simulink library "BasicAircraftDynamicsBlock"  (R2018b)
settings: Solver=VariableStepAuto  StartTime=0.0  StopTime=10.0  RelTol=1e-3
undefined symbols (not defined in the file): ac1dyn_a_ftpss, ac1dyn_con, ac1dyn_E_ft, ac1dyn_h_ft, ac1dyn_N_ft, ac1dyn_phi_rad, ac1dyn_psi_rad, ac1dyn_theta_rad, ac1dyn_v_ftps, ac2dyn_alt0_ft, ac2dyn_lat0_rad, ac2dyn_lon0_rad, DiscIntNeverNeededParam
libraries: simulink x7
settings Model: Creator=BI28030  LastModifiedBy=BI28030

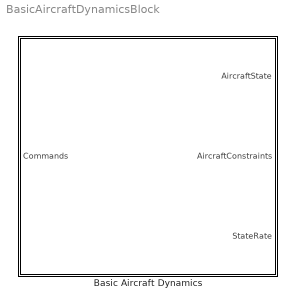
== system BasicAircraftDynamicsBlock ==
  Basic Aircraft Dynamics : Subsystem  mask(Basic Aircraft Dynamic Model){ts_dynamics=.1, v_ftps_0=ac1dyn_v_ftps, N_ft_0=ac1dyn_N_ft, E_ft_0=ac1dyn_E_ft, h_ft_0=ac1dyn_h_ft, psi_rad_0=ac1dyn_psi_rad, theta_rad_0=ac1dyn_theta_rad, phi_rad_0=ac1dyn_phi_rad, a_ftpss_0=ac1dyn_a_ftpss, v_ftps_max=ac1dyn_con.maxAirspeed_ftps, v_ftps_min=ac1dyn_con.minAirspeed_ftps, dv_ftpss_max=ac1dyn_con.maxAcceleration_ftpss, dv_ftpss_min=ac1dyn_con.minAcceleration_ftpss, dh_ftps_max=ac1dyn_con.maxVerticalRate_ftps, dh_ftps_min=ac1dyn_con.minVerticalRate_ftps, q_radps_max=ac1dyn_con.maxPitchRate_radps, phi_rad_max=ac1dyn_con.maxBankAngle_rad, dphi_radps_max=ac1dyn_con.maxRollRate_radps, r_radps_max=ac1dyn_con.maxYawRate_radps, pNUM=ac1dyn_con.dynamicsNumeratorRollRate, pDEN=ac1dyn_con.dynamicsDenominatorRollRate, hNUM=ac1dyn_con.dynamicsNumeratorVerticalRate, hDEN=ac1dyn_con.dynamicsDenominatorVerticalRate, rNUM=ac1dyn_con.dynamicsNumeratorYawRate, rDEN=ac1dyn_con.dynamicsDenominatorYawRate, lat0_rad=ac2dyn_lat0_rad, lon0_rad=ac2dyn_lon0_rad, alt_ft=ac2dyn_alt0_ft}
      mask prompts: ts_dynamics "Dynamics update parameter"; v_ftps_0 "Initial velocity (ft/s)"; N_ft_0 "Initial north position (ft)"; E_ft_0 "Initial east position (ft)"; h_ft_0 "Initial altitude (ft)"; psi_rad_0 "Initial heading (rad)"; theta_rad_0 "Initial pitch angle (rad)"; phi_rad_0 "Initial bank angle (rad)"; a_ftpss_0 "Initial acceleration (ft/s/s)"; v_ftps_max "Maximum airspeed (ft/s)"; v_ftps_min "Minimum airspeed (ft/s)"; dv_ftpss_max "Maximum acceleration (ft/s/s)"; dv_ftpss_min "Miniimum acceleration (ft/s/s)"; dh_ftps_max "Maximum vertical rate (ft/s)"; dh_ftps_min "Minimum vertical rate (ft/s)"; q_radps_max "Maximum pitch rate (rad/s)"; phi_rad_max "Maximum bank angle (rad)"; dphi_radps_max "Maximum roll rate (rad/s)"; r_radps_max "Maximum yaw rate (rad/s)"; pNUM "Roll rate discrete dynamics numerator (2x1)"; pDEN "Roll rate discrete dynamics denominator (1x1)"; hNUM "Vertical rate discrete dynamics numerator (2x1)"; hDEN "Vertical rate discrete dynamics denominator (1x1)"; rNUM "Yaw rate discrete dynamics numerator (2x1)"; rDEN "Yaw rate discrete dynamics denominator (1x1)"; lat0_rad "Latitude of ENU origin (rad)"; lon0_rad "Longitude of ENU origin (rad)"; alt_ft "Height of ENU origin (ft)"
      mask help:
      | Propagates the aircraft dynamics using 6DOF equations of motion.
      |
      | The class Simple6DOF can be used to programmatically set the parameters of Basic Aircraft Dynamics blocks.
      mask Help:
      | Propagates the aircraft dynamics using 6DOF equations of motion.
      | 
      | The class Simple6DOF can be used to programmatically set the parameters of Basic Aircraft Dynamcis blocks.
      mask DialogControl ParameterTabVar0 Prompt: Initial Conditions
      mask DialogControl ParameterTabVar01 Prompt: Constraints
      mask DialogControl ParameterTabVar012 Prompt: ENU Coordinate System

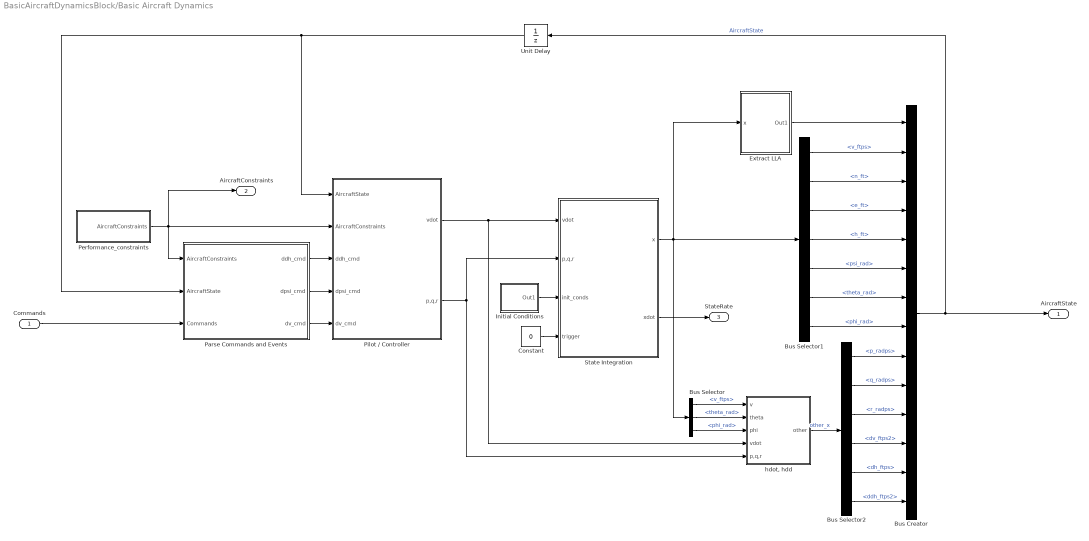
== system BasicAircraftDynamicsBlock/Basic Aircraft Dynamics ==
  Commands : Inport  OutDataTypeStr=Bus: AircraftCommands
  Bus Creator : BusCreator  Inputs=14
  Bus Selector : BusSelector  OutputSignals=v_ftps,theta_rad,phi_rad
  Bus Selector1 : BusSelector  OutputSignals=v_ftps,n_ft,e_ft,h_ft,psi_rad,theta_rad,phi_rad
  Bus Selector2 : BusSelector  OutputSignals=p_radps,q_radps,r_radps,dv_ftps2,dh_ftps,ddh_ftps2
  Constant : Constant  Value=0
  "Extract LLA " : Subsystem  mask{lat0=lat0_rad, lon0=lon0_rad, h0=alt_ft}
      mask prompts: lat0 "ENU latitude origin (rad)"; lon0 "ENU longitude origin (rad)"; h0 "ENU altitude origin (ft)"
  Initial Conditions : Subsystem
  Parse Commands and Events : Subsystem
  Performance_constraints : Subsystem
  Pilot / Controller : Subsystem
  State Integration : Subsystem
  Unit Delay : UnitDelay  SampleTime=-1
  "hdot, hdd" : Subsystem
  AircraftState : Outport  OutDataTypeStr=Bus: AircraftState
  AircraftConstraints : Outport  Port=2  OutDataTypeStr=Bus: AircraftConstraints
  StateRate : Outport  Port=3  OutDataTypeStr=Bus: AircraftStateRate
  wires:
  "Extract LLA "/1(Out1) -> Bus Creator/1
  Initial Conditions/1(Out1) -> State Integration/3(init_conds)
  Bus Selector/1 -> "hdot, hdd"/1(v)  "<v_ftps>"
  Bus Selector/2 -> "hdot, hdd"/2(theta)  "<theta_rad>"
  Bus Selector/3 -> "hdot, hdd"/3(phi)  "<phi_rad>"
  State Integration/1(x) -> Bus Selector/1, "Extract LLA "/1(x), Bus Selector1/1
  Bus Selector1/1 -> Bus Creator/2  "<v_ftps>"
  Bus Selector1/2 -> Bus Creator/3  "<n_ft>"
  Bus Selector1/3 -> Bus Creator/4  "<e_ft>"
  Bus Selector1/4 -> Bus Creator/5  "<h_ft>"
  Bus Selector1/5 -> Bus Creator/6  "<psi_rad>"
  Bus Selector1/6 -> Bus Creator/7  "<theta_rad>"
  Bus Selector1/7 -> Bus Creator/8  "<phi_rad>"
  "hdot, hdd"/1(other) -> Bus Selector2/1  "other_x"
  Bus Selector2/1 -> Bus Creator/9  "<p_radps>"
  Bus Selector2/2 -> Bus Creator/10  "<q_radps>"
  Bus Selector2/3 -> Bus Creator/11  "<r_radps>"
  Bus Selector2/4 -> Bus Creator/12  "<dv_ftps2>"
  Bus Selector2/5 -> Bus Creator/13  "<dh_ftps>"
  Bus Selector2/6 -> Bus Creator/14  "<ddh_ftps2>"
  Bus Creator/1 -> AircraftState/1, Unit Delay/1  "AircraftState"
  Constant/1 -> State Integration/4(trigger)
  Pilot / Controller/1(vdot) -> State Integration/1(vdot), "hdot, hdd"/4(vdot)
  Pilot / Controller/2(p,q,r) -> "hdot, hdd"/5(p,q,r), State Integration/2(p,q,r)
  Performance_constraints/1(AircraftConstraints) -> AircraftConstraints/1, Pilot / Controller/2(AircraftConstraints), Parse Commands and Events/1(AircraftConstraints)
  Commands/1 -> Parse Commands and Events/3(Commands)
  Parse Commands and Events/1(ddh_cmd) -> Pilot / Controller/3(ddh_cmd)
  Parse Commands and Events/2(dpsi_cmd) -> Pilot / Controller/4(dpsi_cmd)
  Parse Commands and Events/3(dv_cmd) -> Pilot / Controller/5(dv_cmd)
  Unit Delay/1 -> Pilot / Controller/1(AircraftState), Parse Commands and Events/2(AircraftState)
  State Integration/2(xdot) -> StateRate/1

== system BasicAircraftDynamicsBlock/Basic Aircraft Dynamics/Extract LLA  ==
  x : Inport
  Bus Creator1 : BusCreator  Inputs=6
  Bus Selector : BusSelector  OutputSignals=e_ft,n_ft,h_ft,v_ftps,psi_rad,theta_rad
  Constant : Constant  Value=lat0_rad
  Constant7 : Constant  Value=lon0_rad
  Constant8 : Constant  Value=alt_ft
  MATLAB Function : MATLAB Function  TreatAsAtomicUnit=on
  Out1 : Outport
  wires:
  Bus Creator1/1 -> Out1/1  "latLonAltState"
  Bus Selector/6 -> MATLAB Function/6(theta_rad)  "<theta_rad>"
  Bus Selector/5 -> MATLAB Function/5(psi_rad)  "<psi_rad>"
  Bus Selector/4 -> MATLAB Function/4(v_ftps)  "<v_ftps>"
  Bus Selector/3 -> MATLAB Function/3(u_ft)  "<h_ft>"
  Bus Selector/2 -> MATLAB Function/2(n_ft)  "<n_ft>"
  Bus Selector/1 -> MATLAB Function/1(e_ft)  "<e_ft>"
  Constant8/1 -> MATLAB Function/9(h0)
  Constant7/1 -> MATLAB Function/8(lon0)
  Constant/1 -> MATLAB Function/7(lat0)
  x/1 -> Bus Selector/1
  MATLAB Function/6(dalt_ftps) -> Bus Creator1/6  "dalt_ftps"
  MATLAB Function/5(alt_ft) -> Bus Creator1/5  "alt_ft"
  MATLAB Function/4(dlon_radps) -> Bus Creator1/4  "dlon_radps"
  MATLAB Function/3(dlat_radps) -> Bus Creator1/3  "dlat_radps"
  MATLAB Function/2(lon_rad) -> Bus Creator1/2  "lon_rad"
  MATLAB Function/1(lat_rad) -> Bus Creator1/1  "lat_rad"

== system BasicAircraftDynamicsBlock/Basic Aircraft Dynamics/Initial Conditions ==
  Bus Creator1 : BusCreator  Inputs=8
  Constant : Constant  Value=v_ftps_0
  Constant1 : Constant  Value=N_ft_0
  Constant2 : Constant  Value=E_ft_0
  Constant3 : Constant  Value=h_ft_0
  Constant4 : Constant  Value=psi_rad_0
  Constant5 : Constant  Value=theta_rad_0
  Constant6 : Constant  Value=phi_rad_0
  Constant7 : Constant  Value=a_ftpss_0
  Out1 : Outport
  wires:
  Constant1/1 -> Bus Creator1/2  "N"
  Constant2/1 -> Bus Creator1/3  "E"
  Constant3/1 -> Bus Creator1/4  "h"
  Constant4/1 -> Bus Creator1/5  "psi"
  Constant5/1 -> Bus Creator1/6  "theta"
  Constant6/1 -> Bus Creator1/7  "phi"
  Constant7/1 -> Bus Creator1/8  "a"
  Constant/1 -> Bus Creator1/1  "v"
  Bus Creator1/1 -> Out1/1

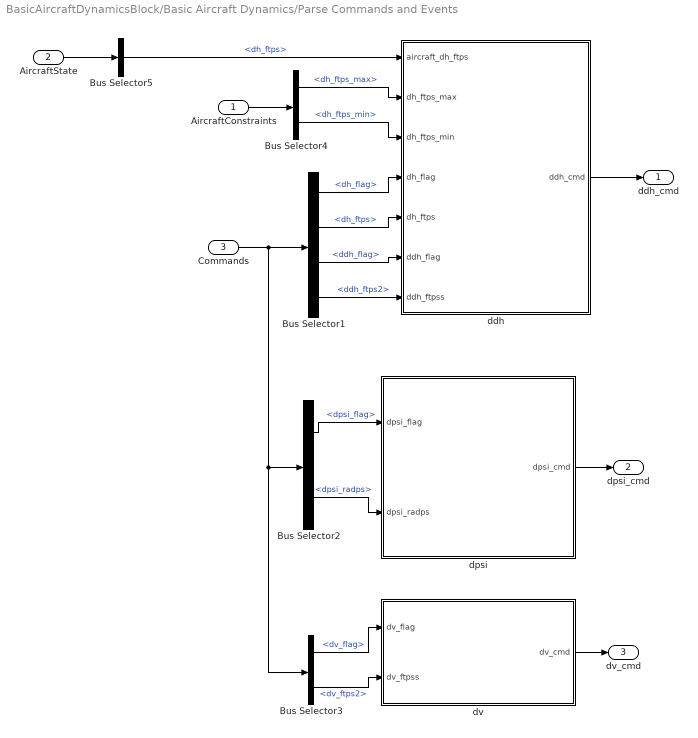
== system BasicAircraftDynamicsBlock/Basic Aircraft Dynamics/Parse Commands and Events ==
  AircraftConstraints : Inport  OutDataTypeStr=Bus: AircraftConstraints
  AircraftState : Inport  Port=2  OutDataTypeStr=Bus: AircraftState
  Commands : Inport  Port=3  OutDataTypeStr=Bus: AircraftCommands
  Bus Selector1 : BusSelector  OutputSignals=dh_flag,dh_ftps,ddh_flag,ddh_ftps2
  Bus Selector2 : BusSelector  OutputSignals=dpsi_flag,dpsi_radps
  Bus Selector3 : BusSelector  OutputSignals=dv_flag,dv_ftps2
  Bus Selector4 : BusSelector  OutputSignals=dh_ftps_max,dh_ftps_min
  Bus Selector5 : BusSelector  OutputSignals=dh_ftps
  ddh : MATLAB Function  TreatAsAtomicUnit=on
  dpsi : MATLAB Function  TreatAsAtomicUnit=on
  dv : MATLAB Function  TreatAsAtomicUnit=on
  ddh_cmd : Outport
  dpsi_cmd : Outport  Port=2
  dv_cmd : Outport  Port=3
  wires:
  dv/1(dv_cmd) -> dv_cmd/1
  dpsi/1(dpsi_cmd) -> dpsi_cmd/1
  ddh/1(ddh_cmd) -> ddh_cmd/1
  Commands/1 -> Bus Selector1/1, Bus Selector2/1, Bus Selector3/1
  Bus Selector1/1 -> ddh/4(dh_flag)  "<dh_flag>"
  Bus Selector1/2 -> ddh/5(dh_ftps)  "<dh_ftps>"
  Bus Selector1/3 -> ddh/6(ddh_flag)  "<ddh_flag>"
  Bus Selector1/4 -> ddh/7(ddh_ftpss)  "<ddh_ftps2>"
  Bus Selector2/2 -> dpsi/2(dpsi_radps)  "<dpsi_radps>"
  Bus Selector3/1 -> dv/1(dv_flag)  "<dv_flag>"
  Bus Selector3/2 -> dv/2(dv_ftpss)  "<dv_ftps2>"
  AircraftConstraints/1 -> Bus Selector4/1
  Bus Selector4/2 -> ddh/3(dh_ftps_min)  "<dh_ftps_min>"
  Bus Selector4/1 -> ddh/2(dh_ftps_max)  "<dh_ftps_max>"
  AircraftState/1 -> Bus Selector5/1
  Bus Selector5/1 -> ddh/1(aircraft_dh_ftps)  "<dh_ftps>"
  Bus Selector2/1 -> dpsi/1(dpsi_flag)  "<dpsi_flag>"

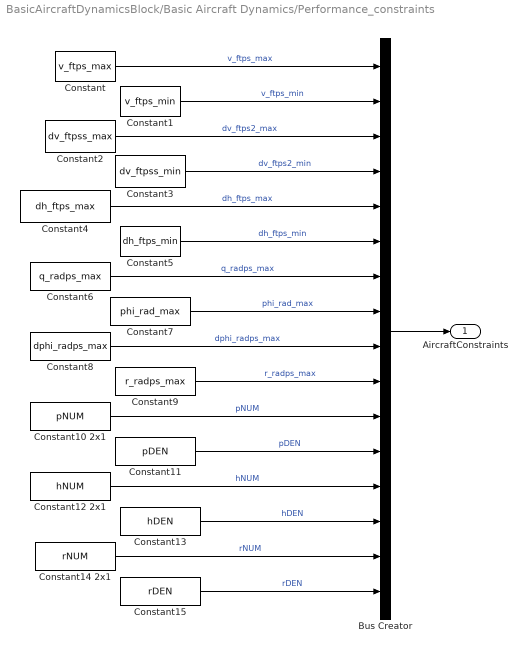
== system BasicAircraftDynamicsBlock/Basic Aircraft Dynamics/Performance_constraints ==
  Bus Creator : BusCreator  Inputs=16
  Constant : Constant  Value=v_ftps_max
  Constant1 : Constant  Value=v_ftps_min
  Constant10 2x1 : Constant  Value=pNUM
  Constant11 : Constant  Value=pDEN
  Constant12 2x1 : Constant  Value=hNUM
  Constant13 : Constant  Value=hDEN
  Constant14 2x1 : Constant  Value=rNUM
  Constant15 : Constant  Value=rDEN
  Constant2 : Constant  Value=dv_ftpss_max
  Constant3 : Constant  Value=dv_ftpss_min
  Constant4 : Constant  Value=dh_ftps_max
  Constant5 : Constant  Value=dh_ftps_min
  Constant6 : Constant  Value=q_radps_max
  Constant7 : Constant  Value=phi_rad_max
  Constant8 : Constant  Value=dphi_radps_max
  Constant9 : Constant  Value=r_radps_max
  AircraftConstraints : Outport  OutDataTypeStr=Bus: AircraftConstraints
  wires:
  Constant10 2x1/1 -> Bus Creator/11  "pNUM"
  Constant12 2x1/1 -> Bus Creator/13  "hNUM"
  Constant14 2x1/1 -> Bus Creator/15  "rNUM"
  Constant8/1 -> Bus Creator/9  "dphi_radps_max"
  Constant7/1 -> Bus Creator/8  "phi_rad_max"
  Constant6/1 -> Bus Creator/7  "q_radps_max"
  Constant5/1 -> Bus Creator/6  "dh_ftps_min"
  Constant4/1 -> Bus Creator/5  "dh_ftps_max"
  Constant3/1 -> Bus Creator/4  "dv_ftps2_min"
  Constant2/1 -> Bus Creator/3  "dv_ftps2_max"
  Constant1/1 -> Bus Creator/2  "v_ftps_min"
  Constant/1 -> Bus Creator/1  "v_ftps_max"
  Bus Creator/1 -> AircraftConstraints/1
  Constant15/1 -> Bus Creator/16  "rDEN"
  Constant13/1 -> Bus Creator/14  "hDEN"
  Constant11/1 -> Bus Creator/12  "pDEN"
  Constant9/1 -> Bus Creator/10  "r_radps_max"

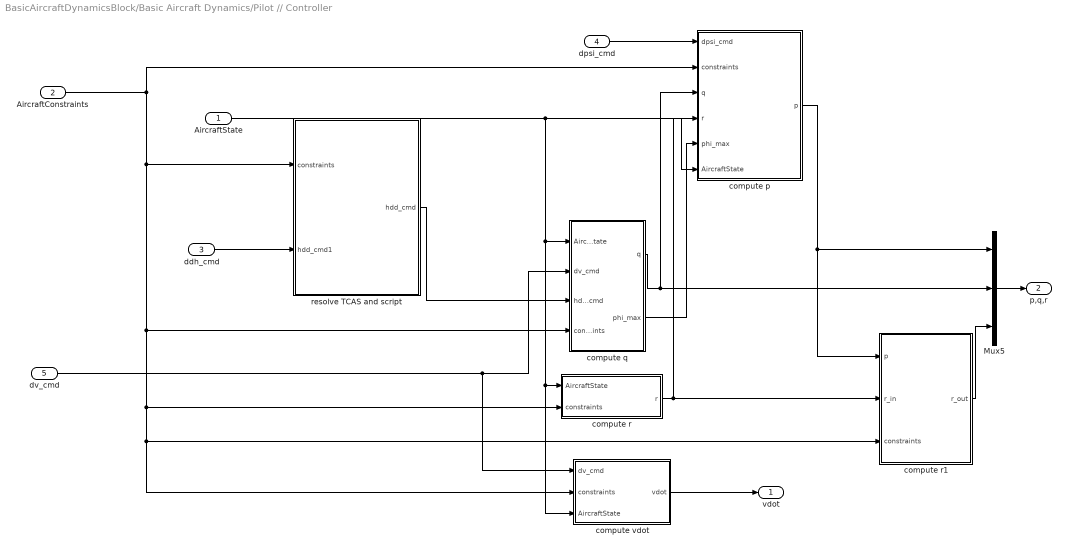
== system BasicAircraftDynamicsBlock/Basic Aircraft Dynamics/Pilot // Controller ==
  AircraftState : Inport  OutDataTypeStr=Bus: AircraftState
  AircraftConstraints : Inport  Port=2
  ddh_cmd : Inport  Port=3
  dpsi_cmd : Inport  Port=4
  dv_cmd : Inport  Port=5
  " compute vdot" : Subsystem
  Mux5 : Mux  Inputs=3
  compute p : Subsystem
  compute q : Subsystem
  compute r : Subsystem
  compute r1 : Subsystem
  resolve TCAS and script : Subsystem
  vdot : Outport
  p,q,r : Outport  Port=2
  wires:
  compute r1/1(r_out) -> Mux5/3
  compute p/1(p) -> Mux5/1, compute r1/1(p)
  resolve TCAS and script/1(hdd_cmd) -> compute q/3(hdd_cmd)
  compute r/1(r) -> compute r1/2(r_in), compute p/4(r)
  compute q/1(q) -> compute p/3(q), Mux5/2
  " compute vdot"/1(vdot) -> vdot/1
  Mux5/1 -> p,q,r/1
  compute q/2(phi_max) -> compute p/5(phi_max)
  ddh_cmd/1 -> resolve TCAS and script/2(hdd_cmd1)
  AircraftState/1 -> compute p/6(AircraftState), compute q/1(AircraftState), compute r/1(AircraftState), " compute vdot"/3(AircraftState)
  AircraftConstraints/1 -> resolve TCAS and script/1(constraints), compute q/4(constraints), compute r/2(constraints), " compute vdot"/2(constraints), compute r1/3(constraints), compute p/2(constraints)
  dv_cmd/1 -> compute q/2(dv_cmd), " compute vdot"/1(dv_cmd)
  dpsi_cmd/1 -> compute p/1(dpsi_cmd)

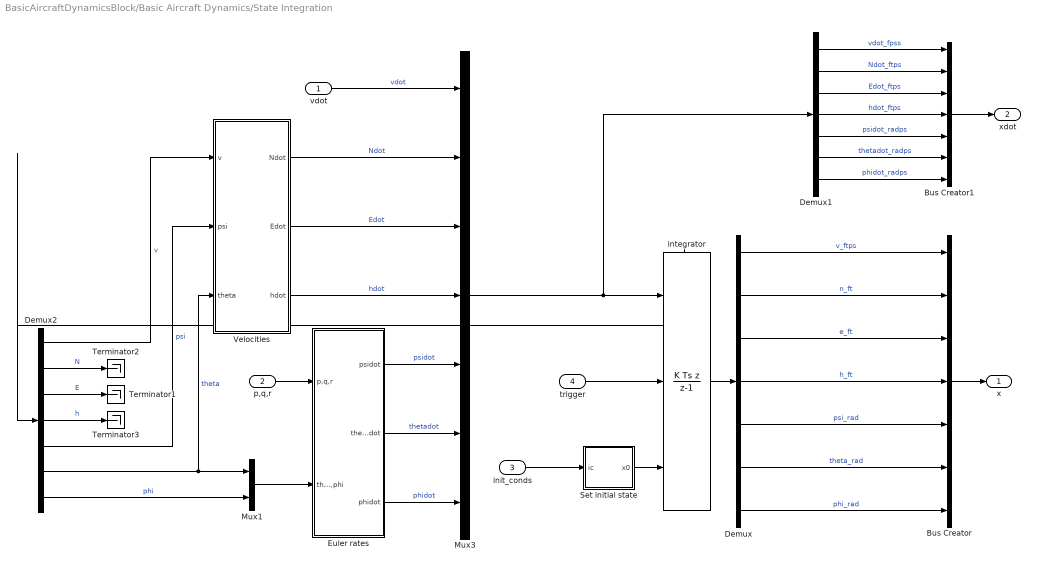
== system BasicAircraftDynamicsBlock/Basic Aircraft Dynamics/State Integration ==
  vdot : Inport
  p,q,r : Inport  Port=2
  init_conds : Inport  Port=3
  trigger : Inport  Port=4
  Bus Creator : BusCreator  Inputs=7
  Bus Creator1 : BusCreator  Inputs=7  OutDataTypeStr=Bus: AircraftStateRate
  Demux : Demux  Outputs=7
  Demux1 : Demux  Outputs=7
  Demux2 : Demux  Outputs=7
  Euler rates : Subsystem
  Mux1 : Mux  Inputs=2
  Mux3 : Mux  Inputs=7
  Set initial state : Subsystem
  Terminator1 : Terminator
  Terminator2 : Terminator
  Terminator3 : Terminator
  Velocities : Subsystem
  integrator : DiscreteIntegrator  IntegratorMethod=Integration: Backward Euler  ExternalReset=rising  InitialConditionSource=external  InitialCondition=200  SampleTime=ts_dynamics  ShowStatePort=on  ICPrevOutput=DiscIntNeverNeededParam  ICPrevScaledInput=DiscIntNeverNeededParam
  x : Outport
  xdot : Outport  Port=2  OutDataTypeStr=Bus: AircraftStateRate
  wires:
  integrator/State -> Demux2/1
  Mux3/1 -> Demux1/1, integrator/1
  Demux2/7 -> Mux1/2  "phi"
  Euler rates/3(phidot) -> Mux3/7  "phidot"
  Euler rates/2(thetadot) -> Mux3/6  "thetadot"
  Euler rates/1(psidot) -> Mux3/5  "psidot"
  Demux2/6 -> Mux1/1, Velocities/3(theta)  "theta"
  Demux2/5 -> Velocities/2(psi)  "psi"
  Demux2/1 -> Velocities/1(v)  "v"
  Velocities/3(hdot) -> Mux3/4  "hdot"
  Velocities/2(Edot) -> Mux3/3  "Edot"
  Velocities/1(Ndot) -> Mux3/2  "Ndot"
  Demux2/3 -> Terminator1/1  "E"
  Demux2/2 -> Terminator2/1  "N"
  p,q,r/1 -> Euler rates/1(p,q,r)
  Mux1/1 -> Euler rates/2(theta,phi)
  Set initial state/1(x0) -> integrator/3
  init_conds/1 -> Set initial state/1(ic)
  Bus Creator/1 -> x/1
  Demux/4 -> Bus Creator/4  "h_ft"
  Demux2/4 -> Terminator3/1  "h"
  vdot/1 -> Mux3/1  "vdot"
  Demux/2 -> Bus Creator/2  "n_ft"
  Demux/3 -> Bus Creator/3  "e_ft"
  Demux/5 -> Bus Creator/5  "psi_rad"
  Demux/6 -> Bus Creator/6  "theta_rad"
  integrator/1 -> Demux/1
  Demux/7 -> Bus Creator/7  "phi_rad"
  Demux/1 -> Bus Creator/1  "v_ftps"
  trigger/1 -> integrator/2
  Bus Creator1/1 -> xdot/1
  Demux1/1 -> Bus Creator1/1  "vdot_fpss"
  Demux1/2 -> Bus Creator1/2  "Ndot_ftps"
  Demux1/3 -> Bus Creator1/3  "Edot_ftps"
  Demux1/4 -> Bus Creator1/4  "hdot_ftps"
  Demux1/5 -> Bus Creator1/5  "psidot_radps"
  Demux1/6 -> Bus Creator1/6  "thetadot_radps"
  Demux1/7 -> Bus Creator1/7  "phidot_radps"

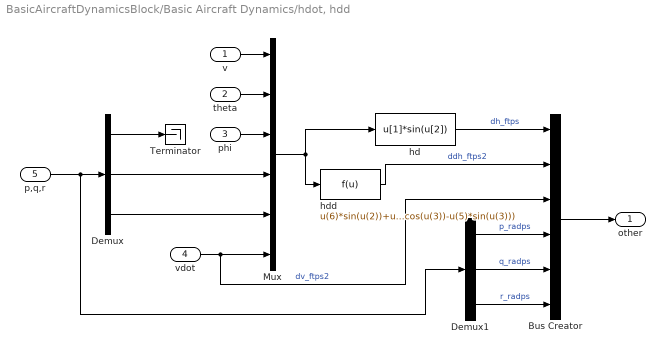
== system BasicAircraftDynamicsBlock/Basic Aircraft Dynamics/hdot, hdd ==
  v : Inport
  theta : Inport  Port=2
  phi : Inport  Port=3
  vdot : Inport  Port=4
  p,q,r : Inport  Port=5
  Bus Creator : BusCreator  Inputs=6
  Demux : Demux  Outputs=3
  Demux1 : Demux  Outputs=3
  Mux : Mux  Inputs=6
  Terminator : Terminator
  hd : Fcn  Expr=u[1]*sin(u[2])
  hdd : Fcn  Expr=u(6)*sin(u(2))+u(1)*cos(u(2))*(u(4)*cos(u(3))-u(5)*sin(u(3)))
  other : Outport
  wires:
  p,q,r/1 -> Demux/1, Demux1/1
  Demux/1 -> Terminator/1
  v/1 -> Mux/1
  theta/1 -> Mux/2
  Mux/1 -> hdd/1, hd/1
  Bus Creator/1 -> other/1
  hdd/1 -> Bus Creator/2  "ddh_ftps2"
  hd/1 -> Bus Creator/1  "dh_ftps"
  phi/1 -> Mux/3
  Demux/2 -> Mux/4
  Demux/3 -> Mux/5
  vdot/1 -> Mux/6, Bus Creator/3  "dv_ftps2"
  Demux1/1 -> Bus Creator/4  "p_radps"
  Demux1/2 -> Bus Creator/5  "q_radps"
  Demux1/3 -> Bus Creator/6  "r_radps"

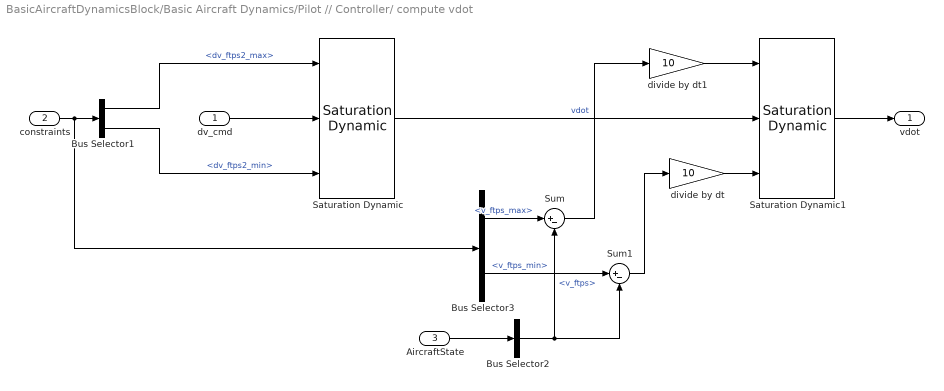
== system BasicAircraftDynamicsBlock/Basic Aircraft Dynamics/Pilot // Controller/ compute vdot ==
  dv_cmd : Inport
  constraints : Inport  Port=2
  AircraftState : Inport  Port=3  OutDataTypeStr=Bus: AircraftState
  Bus Selector1 : BusSelector  OutputSignals=dv_ftps2_max,dv_ftps2_min
  Bus Selector2 : BusSelector  OutputSignals=v_ftps
  Bus Selector3 : BusSelector  OutputSignals=v_ftps_max,v_ftps_min
  Saturation Dynamic : simulink/Discontinuities/Saturation Dynamic  OutMin=[]  OutMax=[]  OutDataTypeStr=Inherit: Same as second input  OutDataType=sfix(16)  OutScaling=2^-10  DoSatur=off
  Saturation Dynamic1 : simulink/Discontinuities/Saturation Dynamic  OutMin=[]  OutMax=[]  OutDataTypeStr=Inherit: Same as second input  OutDataType=sfix(16)  OutScaling=2^-10  DoSatur=off
  Sum : Sum  Inputs=|+-
  Sum1 : Sum  Inputs=|+-
  divide by dt : Gain  Gain=10
  divide by dt1 : Gain  Gain=10
  vdot : Outport
  wires:
  Sum1/1 -> divide by dt/1
  Bus Selector3/2 -> Sum1/1  "<v_ftps_min>"
  Sum/1 -> divide by dt1/1
  Bus Selector2/1 -> Sum1/2, Sum/2  "<v_ftps>"
  Bus Selector3/1 -> Sum/1  "<v_ftps_max>"
  divide by dt/1 -> Saturation Dynamic1/3
  divide by dt1/1 -> Saturation Dynamic1/1
  Saturation Dynamic1/1 -> vdot/1
  AircraftState/1 -> Bus Selector2/1
  Saturation Dynamic/1 -> Saturation Dynamic1/2  "vdot"
  dv_cmd/1 -> Saturation Dynamic/2
  constraints/1 -> Bus Selector3/1, Bus Selector1/1
  Bus Selector1/2 -> Saturation Dynamic/3  "<dv_ftps2_min>"
  Bus Selector1/1 -> Saturation Dynamic/1  "<dv_ftps2_max>"

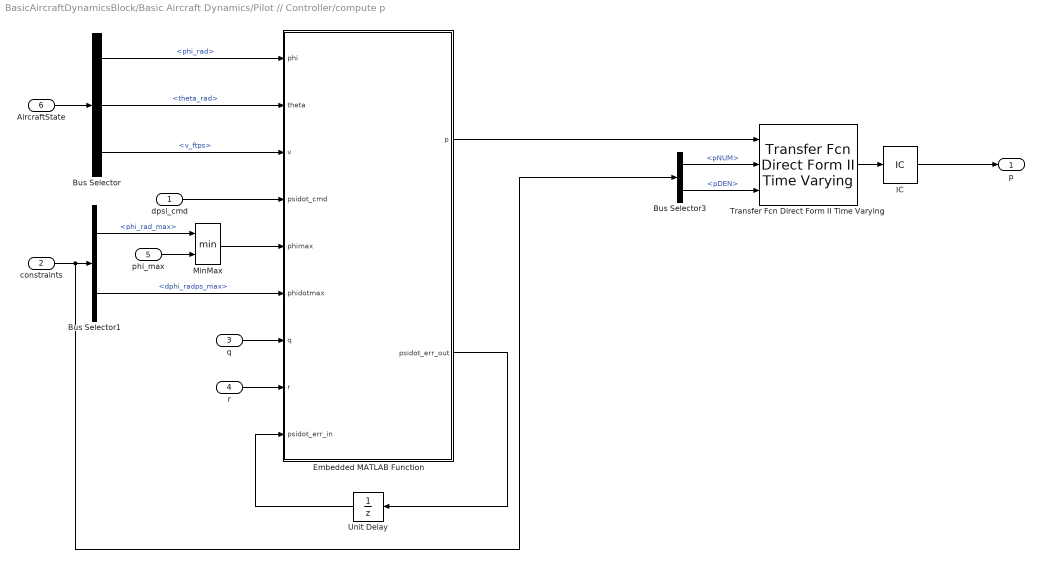
== system BasicAircraftDynamicsBlock/Basic Aircraft Dynamics/Pilot // Controller/compute p ==
  dpsi_cmd : Inport
  constraints : Inport  Port=2
  q : Inport  Port=3
  r : Inport  Port=4
  phi_max : Inport  Port=5
  AircraftState : Inport  Port=6  OutDataTypeStr=Bus: AircraftState
  Bus Selector : BusSelector  OutputSignals=phi_rad,theta_rad,v_ftps
  Bus Selector1 : BusSelector  OutputSignals=phi_rad_max,dphi_radps_max
  Bus Selector3 : BusSelector  OutputSignals=pNUM,pDEN
  Embedded MATLAB Function : MATLAB Function  TreatAsAtomicUnit=on
  IC : InitialCondition  Value=0  SampleTime=ts_dynamics
  MinMax : MinMax  Inputs=2  SampleTime=ts_dynamics
  Transfer Fcn Direct Form II Time Varying : simulink/Additional Math & Discrete/Additional Discrete/Transfer Fcn Direct Form II Time Varying  vinit=0.0  DoSatur=off
      settings: SourceProductName=Simulink  SourceProductBaseCode=SL
  Unit Delay : UnitDelay  SampleTime=ts_dynamics
  p : Outport
  wires:
  Bus Selector3/2 -> Transfer Fcn Direct Form II Time Varying/3  "<pDEN>"
  Bus Selector3/1 -> Transfer Fcn Direct Form II Time Varying/2  "<pNUM>"
  Embedded MATLAB Function/1(p) -> Transfer Fcn Direct Form II Time Varying/1
  IC/1 -> p/1
  Transfer Fcn Direct Form II Time Varying/1 -> IC/1
  Unit Delay/1 -> Embedded MATLAB Function/9(psidot_err_in)
  Embedded MATLAB Function/2(psidot_err_out) -> Unit Delay/1
  Bus Selector1/2 -> Embedded MATLAB Function/6(phidotmax)  "<dphi_radps_max>"
  r/1 -> Embedded MATLAB Function/8(r)
  q/1 -> Embedded MATLAB Function/7(q)
  Bus Selector/3 -> Embedded MATLAB Function/3(v)  "<v_ftps>"
  Bus Selector/2 -> Embedded MATLAB Function/2(theta)  "<theta_rad>"
  Bus Selector/1 -> Embedded MATLAB Function/1(phi)  "<phi_rad>"
  AircraftState/1 -> Bus Selector/1
  dpsi_cmd/1 -> Embedded MATLAB Function/4(psidot_cmd)
  constraints/1 -> Bus Selector3/1, Bus Selector1/1
  phi_max/1 -> MinMax/2
  Bus Selector1/1 -> MinMax/1  "<phi_rad_max>"
  MinMax/1 -> Embedded MATLAB Function/5(phimax)

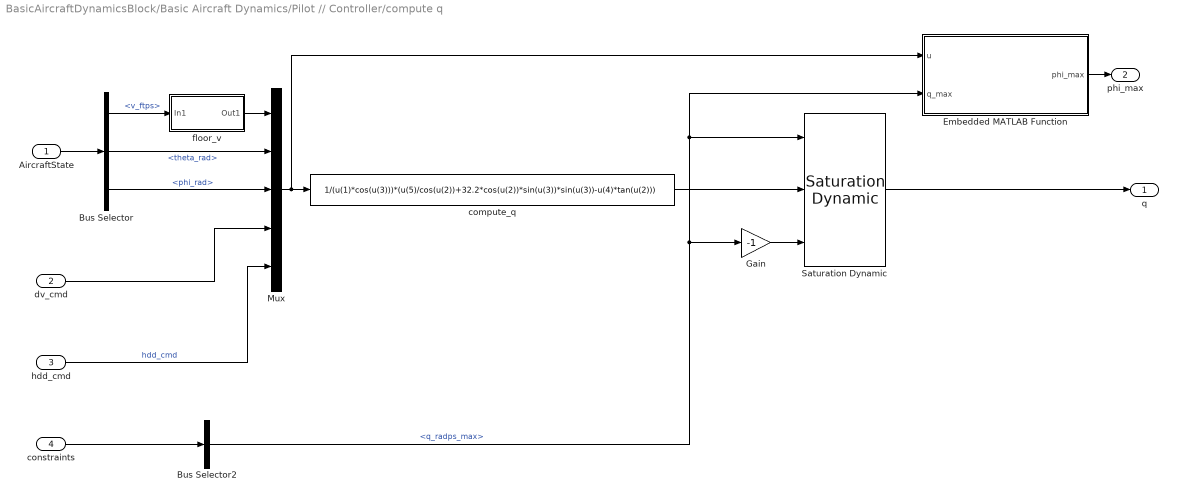
== system BasicAircraftDynamicsBlock/Basic Aircraft Dynamics/Pilot // Controller/compute q ==
  AircraftState : Inport  OutDataTypeStr=Bus: AircraftState
  dv_cmd : Inport  Port=2
  hdd_cmd : Inport  Port=3
  constraints : Inport  Port=4
  Bus Selector : BusSelector  OutputSignals=v_ftps,theta_rad,phi_rad
  Bus Selector2 : BusSelector  OutputSignals=q_radps_max
  Embedded MATLAB Function : MATLAB Function  TreatAsAtomicUnit=on
  Gain : Gain  Gain=-1  SampleTime=ts_dynamics
  Mux : Mux  Inputs=5
  Saturation Dynamic : simulink/Discontinuities/Saturation Dynamic  OutMin=[]  OutMax=[]  OutDataTypeStr=Inherit: Same as second input  OutDataType=sfix(16)  OutScaling=2^-10  DoSatur=off
  compute_q : Fcn  Expr=1/(u(1)*cos(u(3)))*(u(5)/cos(u(2))+32.2*cos(u(2))*sin(u(3))*sin(u(3))-u(4)*tan(u(2)))  SampleTime=ts_dynamics
  floor_v : Subsystem
  q : Outport
  phi_max : Outport  Port=2
  wires:
  floor_v/1(Out1) -> Mux/1
  AircraftState/1 -> Bus Selector/1
  Bus Selector/1 -> floor_v/1(In1)  "<v_ftps>"
  Bus Selector/2 -> Mux/2  "<theta_rad>"
  Bus Selector/3 -> Mux/3  "<phi_rad>"
  Mux/1 -> compute_q/1, Embedded MATLAB Function/1(u)
  dv_cmd/1 -> Mux/4
  hdd_cmd/1 -> Mux/5  "hdd_cmd"
  constraints/1 -> Bus Selector2/1
  Bus Selector2/1 -> Gain/1, Saturation Dynamic/1, Embedded MATLAB Function/2(q_max)  "<q_radps_max>"
  compute_q/1 -> Saturation Dynamic/2
  Gain/1 -> Saturation Dynamic/3
  Embedded MATLAB Function/1(phi_max) -> phi_max/1
  Saturation Dynamic/1 -> q/1

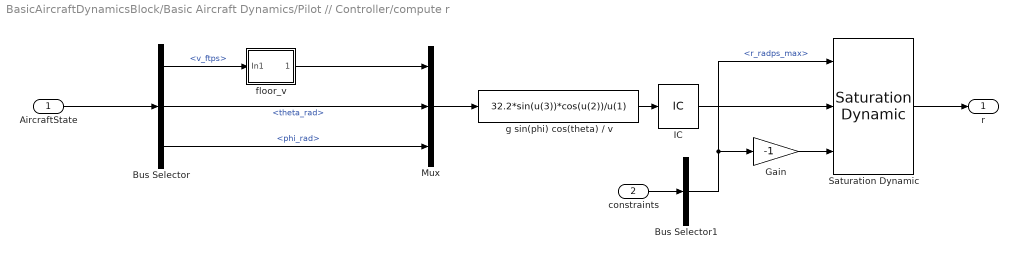
== system BasicAircraftDynamicsBlock/Basic Aircraft Dynamics/Pilot // Controller/compute r ==
  AircraftState : Inport  OutDataTypeStr=Bus: AircraftState
  constraints : Inport  Port=2
  Bus Selector : BusSelector  OutputSignals=v_ftps,theta_rad,phi_rad
  Bus Selector1 : BusSelector  OutputSignals=r_radps_max
  Gain : Gain  Gain=-1
  IC : InitialCondition  Value=0
  Mux : Mux  Inputs=3
  Saturation Dynamic : simulink/Discontinuities/Saturation Dynamic  OutMin=[]  OutMax=[]  OutDataTypeStr=Inherit: Same as second input  OutDataType=sfix(16)  OutScaling=2^-10  DoSatur=off
  floor_v : Subsystem
  g sin(phi) cos(theta) / v : Fcn  Expr=32.2*sin(u(3))*cos(u(2))/u(1)
  r : Outport
  wires:
  Gain/1 -> Saturation Dynamic/3
  Bus Selector1/1 -> Saturation Dynamic/1, Gain/1  "<r_radps_max>"
  constraints/1 -> Bus Selector1/1
  Saturation Dynamic/1 -> r/1
  IC/1 -> Saturation Dynamic/2
  floor_v/1(Out1) -> Mux/1
  AircraftState/1 -> Bus Selector/1
  Bus Selector/1 -> floor_v/1(In1)  "<v_ftps>"
  Bus Selector/2 -> Mux/2  "<theta_rad>"
  Bus Selector/3 -> Mux/3  "<phi_rad>"
  Mux/1 -> g sin(phi) cos(theta) / v/1
  g sin(phi) cos(theta) / v/1 -> IC/1

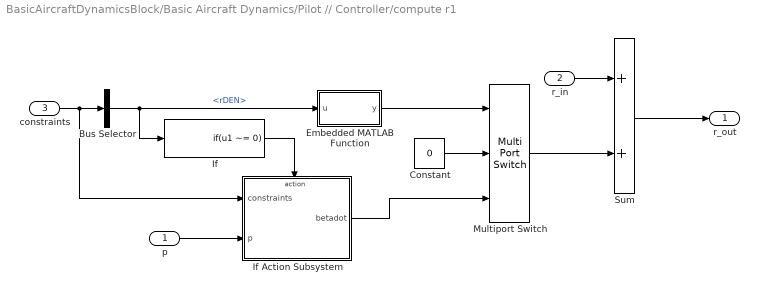
== system BasicAircraftDynamicsBlock/Basic Aircraft Dynamics/Pilot // Controller/compute r1 ==
  p : Inport
  r_in : Inport  Port=2
  constraints : Inport  Port=3
  Bus Selector : BusSelector  OutputSignals=rDEN
  Constant : Constant  Value=0
  Embedded MATLAB Function : MATLAB Function  TreatAsAtomicUnit=on
  If : If  IfExpression=u1 ~= 0  ShowElse=off
  If Action Subsystem : Subsystem  TreatAsAtomicUnit=on
  Multiport Switch : MultiPortSwitch  Inputs=2
  Sum : Sum
  r_out : Outport
  wires:
  If Action Subsystem/1(betadot) -> Multiport Switch/3
  p/1 -> If Action Subsystem/2(p)
  If/1 -> If Action Subsystem/Action
  Bus Selector/1 -> If/1, Embedded MATLAB Function/1(u)  "<rDEN>"
  constraints/1 -> If Action Subsystem/1(constraints), Bus Selector/1
  r_in/1 -> Sum/1
  Constant/1 -> Multiport Switch/2
  Multiport Switch/1 -> Sum/2
  Sum/1 -> r_out/1
  Embedded MATLAB Function/1(y) -> Multiport Switch/1

== system BasicAircraftDynamicsBlock/Basic Aircraft Dynamics/Pilot // Controller/resolve TCAS and script ==
  constraints : Inport
  hdd_cmd1 : Inport  Port=2
  Bus Selector3 : BusSelector  OutputSignals=hNUM,hDEN
  Transfer Fcn Direct Form II Time Varying : simulink/Additional Math & Discrete/Additional Discrete/Transfer Fcn Direct Form II Time Varying  vinit=0.0  DoSatur=off
      settings: SourceProductName=Simulink  SourceProductBaseCode=SL
  hdd_cmd : Outport
  wires:
  Bus Selector3/2 -> Transfer Fcn Direct Form II Time Varying/3  "<hDEN>"
  Bus Selector3/1 -> Transfer Fcn Direct Form II Time Varying/2  "<hNUM>"
  Transfer Fcn Direct Form II Time Varying/1 -> hdd_cmd/1
  constraints/1 -> Bus Selector3/1
  hdd_cmd1/1 -> Transfer Fcn Direct Form II Time Varying/1

== system BasicAircraftDynamicsBlock/Basic Aircraft Dynamics/State Integration/Euler rates ==
  p,q,r : Inport
  theta,phi : Inport  Port=2
  Compute phidot : Fcn  Expr=u(1)+u(2)*sin(u(5))*tan(u(4))+u(3)*cos(u(5))*tan(u(4))
  Compute psidot : Fcn  Expr=u(2)*sin(u(5))/cos(u(4))+u(3)*cos(u(5))/cos(u(4))
  Compute thetadot : Fcn  Expr=u(2)*cos(u(5))-u(3)*sin(u(5))
  Mux : Mux  Inputs=2
  psidot : Outport
  thetadot : Outport  Port=2
  phidot : Outport  Port=3
  wires:
  Compute phidot/1 -> phidot/1
  Compute thetadot/1 -> thetadot/1
  Compute psidot/1 -> psidot/1
  Mux/1 -> Compute psidot/1, Compute thetadot/1, Compute phidot/1
  theta,phi/1 -> Mux/2
  p,q,r/1 -> Mux/1

== system BasicAircraftDynamicsBlock/Basic Aircraft Dynamics/State Integration/Set initial state ==
  ic : Inport
  Bus Selector : BusSelector  OutputSignals=v,N,E,h,psi,theta,phi
  Mux : Mux  Inputs=7
  x0 : Outport
  wires:
  Bus Selector/7 -> Mux/7  "<phi>"
  ic/1 -> Bus Selector/1
  Bus Selector/6 -> Mux/6  "<theta>"
  Bus Selector/5 -> Mux/5  "<psi>"
  Bus Selector/4 -> Mux/4  "<h>"
  Bus Selector/3 -> Mux/3  "<E>"
  Bus Selector/2 -> Mux/2  "<N>"
  Mux/1 -> x0/1
  Bus Selector/1 -> Mux/1  "<v>"

== system BasicAircraftDynamicsBlock/Basic Aircraft Dynamics/State Integration/Velocities ==
  v : Inport
  psi : Inport  Port=2
  theta : Inport  Port=3
  Compute Edot : Fcn  Expr=u(1)*cos(u(2))*sin(u(3))
  Compute Ndot : Fcn  Expr=u(1)*cos(u(2))*cos(u(3))
  Compute hdot : Fcn  Expr=u(1)*sin(u(2))
  Mux : Mux  Inputs=3
  Ndot : Outport
  Edot : Outport  Port=2
  hdot : Outport  Port=3
  wires:
  Compute Ndot/1 -> Ndot/1
  Compute Edot/1 -> Edot/1
  Compute hdot/1 -> hdot/1
  Mux/1 -> Compute Edot/1, Compute hdot/1, Compute Ndot/1
  psi/1 -> Mux/3
  v/1 -> Mux/1
  theta/1 -> Mux/2

== system BasicAircraftDynamicsBlock/Basic Aircraft Dynamics/Pilot // Controller/compute q/floor_v ==
  In1 : Inport
  Constant : Constant
  MinMax : MinMax  Function=max  Inputs=2  SampleTime=ts_dynamics
  Out1 : Outport
  wires:
  MinMax/1 -> Out1/1
  In1/1 -> MinMax/2
  Constant/1 -> MinMax/1

== system BasicAircraftDynamicsBlock/Basic Aircraft Dynamics/Pilot // Controller/compute r/floor_v ==
  In1 : Inport
  Constant : Constant
  MinMax : MinMax  Function=max  Inputs=2  SampleTime=ts_dynamics
  Out1 : Outport
  wires:
  MinMax/1 -> Out1/1
  In1/1 -> MinMax/2
  Constant/1 -> MinMax/1

== system BasicAircraftDynamicsBlock/Basic Aircraft Dynamics/Pilot // Controller/compute r1/If Action Subsystem ==
  constraints : Inport
  p : Inport  Port=2
  Action Port : ActionPort  PropagateVarSize=During execution
  Bus Selector : BusSelector  OutputSignals=rNUM,rDEN
  Transfer Fcn Direct Form II Time Varying : simulink/Additional Math & Discrete/Additional Discrete/Transfer Fcn Direct Form II Time Varying  vinit=0.0  DoSatur=off
      settings: SourceProductName=Simulink  SourceProductBaseCode=SL
  betadot : Outport
  wires:
  Bus Selector/2 -> Transfer Fcn Direct Form II Time Varying/3  "<rDEN>"
  Bus Selector/1 -> Transfer Fcn Direct Form II Time Varying/2  "<rNUM>"
  constraints/1 -> Bus Selector/1
  Transfer Fcn Direct Form II Time Varying/1 -> betadot/1
  p/1 -> Transfer Fcn Direct Form II Time Varying/1

== matlab function BasicAircraftDynamicsBlock/Basic Aircraft Dynamics/Extract LLA /MATLAB Function ==
  data: e_ft input; n_ft input; u_ft input; v_ftps input; psi_rad input; theta_rad input; lat0 input; lat_rad output; lon0 input; h0 input; lon_rad output; dlat_radps output; dlon_radps output; alt_ft output; dalt_ftps output
function [lat_rad,lon_rad,dlat_radps,dlon_radps,alt_ft,dalt_ftps] = convertToLLA(e_ft,n_ft,u_ft,v_ftps,psi_rad,theta_rad,lat0,lon0,h0)
%#codegen

% WGS-84 ellipsoid constants
a = 2.09256*10^7;          %Semi-major axis (meters)
f = 1.0/298.257223563;  %Flattening
ecc_sq = f*(2.0-f);        %Eccentricity^2


% Ellipsoidal "radius"
er = a./sqrt(1-ecc_sq.*sin(lat0).^2);


% ECEF coordinates
x0 = (er + h0)*cos(lat0)*cos(lon0);
y0 = (er + h0)*cos(lat0)*sin(lon0);
z0 = (er.*(1-ecc_sq) + h0)*sin(lat0);


%% Rotation Matrix
posECEF0 = [x0;y0;z0];
% Compute the local Up unit vector
vHatU = posECEF0;
vHatU(3) = vHatU(3) ./ ((1-f)^2);
vHatU = vHatU ./ norm(vHatU);

% Compute the projection onto the local Up vector
pU = vHatU * vHatU';

% Compute the projection onto the local Tangent plane
pT = eye(size(pU)) - pU;

% Compute the local North unit vector
vHatZ = [0;0;1];
vHatN = pT * vHatZ;
vHatN = vHatN ./ norm(vHatN);

% Compute the local East unit vector
vHatE = cross(vHatN,vHatU);

% Compute ENU rotation matrix
rotMatENU = zeros(3,3);
rotMatENU(:,1) = vHatE;
rotMatENU(:,2) = vHatN;
rotMatENU(:,3) = vHatU;

tPosECEF = rotMatENU*[e_ft;n_ft;u_ft] + [x0;y0;z0];


%% ECEF to LLA
% WGS-84 derived parameters
b = (1-f).*a;                       %Semi-minor axis (meters)
ecc1_sq = (a.^2 - b.^2)./(a.^2);    %First eccentricity squared
ecc2_sq = (a.^2 - b.^2)./(b.^2);    %Second eccentricity squared


% Length of position vector in equatorial plane
rho = sqrt(tPosECEF(1).^2 + tPosECEF(2).^2);

% Auxillary angle
theta = atan( (tPosECEF(3).*a)./(rho.*b) );

lon_rad = atan2(tPosECEF(2),tPosECEF(1));
lat_rad = atan( (tPosECEF(3) + ecc2_sq.*b.*(sin(theta)).^3)./(rho - ecc1_sq.*a.*(cos(theta)).^3) );

ewRadCurv = a./sqrt(1-ecc1_sq.*sin(lat_rad).^2);

alt_ft = (rho./cos(lat_rad)) - ewRadCurv;


%% Velocities - Project 1 sec into future and use to estimate
dalt_ftps = v_ftps*sin(theta_rad); % Assume about the same


tPosECEF_1sec = rotMatENU*[e_ft+v_ftps*sin(theta_rad)*sin(psi_rad);...
                           n_ft+v_ftps*sin(theta_rad)*cos(psi_rad);...
                           u_ft] + ...
                           [x0;y0;z0];

% Length of position vector in equatorial plane
rho = sqrt(tPosECEF_1sec(1).^2 + tPosECEF_1sec(2).^2);

% Auxillary angle
theta = atan( (tPosECEF_1sec(3).*a)./(rho.*b) );

lon_rad_1sec = atan2(tPosECEF_1sec(2),tPosECEF_1sec(1));
lat_rad_1sec = atan( (tPosECEF_1sec(3) + ecc2_sq.*b.*(sin(theta)).^3)./(rho - ecc1_sq.*a.*(cos(theta)).^3) );

dlat_radps = lat_rad_1sec - lat_rad;
dlon_radps = lon_rad_1sec - lon_rad;
end

== matlab function BasicAircraftDynamicsBlock/Basic Aircraft Dynamics/Parse Commands and Events/ddh ==
  data: aircraft_dh_ftps input; dh_ftps_max input; dh_ftps_min input; ddh_cmd output; dh_flag input; dh_ftps input; ddh_flag input; ddh_ftpss input
function ddh_cmd = calc_ddh(aircraft_dh_ftps, dh_ftps_max, dh_ftps_min, ...
    dh_flag, dh_ftps, ddh_flag, ddh_ftpss)
%#codegen

% Select appropriate Command
if ddh_flag && ~dh_flag
    ddh_cmd = ddh_ftpss;
    return;
elseif dh_flag && ~ddh_flag
    dh_cmd = dh_ftps;
else
    dh_cmd = aircraft_dh_ftps; % nothing commanded
end

% Limit Vertical Rate
dh_cmd = max( min( dh_ftps_max, dh_cmd ), dh_ftps_min );


ddh_cmd = (dh_cmd-aircraft_dh_ftps)/.1;

== matlab function BasicAircraftDynamicsBlock/Basic Aircraft Dynamics/Parse Commands and Events/dpsi ==
  data: dpsi_cmd output; dpsi_flag input; dpsi_radps input
function dpsi_cmd = calc_dpsi(dpsi_flag, dpsi_radps)
%#codegen

if dpsi_flag 
    dpsi_cmd = dpsi_radps;
else
    dpsi_cmd = 0;
end

== matlab function BasicAircraftDynamicsBlock/Basic Aircraft Dynamics/Parse Commands and Events/dv ==
  data: dv_cmd output; dv_flag input; dv_ftpss input
function dv_cmd= calc_dv(dv_flag, dv_ftpss)
%#codegen

if dv_flag
    dv_cmd = dv_ftpss;
else
    dv_cmd = 0;
end

== matlab function BasicAircraftDynamicsBlock/Basic Aircraft Dynamics/Pilot // Controller/compute p/Embedded MATLAB Function ==
  data: phi input; p output; theta input; v input; psidot_cmd input; phimax input; phidotmax input; q input; r input; psidot_err_out output double size=1; psidot_err_in input double size=1
function [p, psidot_err_out] = compute_p(phi, theta, v, psidot_cmd, phimax, ...
    phidotmax, q, r, psidot_err_in)
% This block supports an embeddable subset of the MATLAB language.
% See the help menu for details. 

phi_cmd0 = atan(psidot_cmd*v/32.2);



psidot_if_no_change = (q*sin(phi)+r*cos(phi))/cos(theta);

dpsidot = psidot_cmd - psidot_if_no_change;
psidot_err_out = psidot_err_in + dpsidot;

%p = 0*(phi_cmd0 - phi) + 20*dpsidot + 0.01*psidot_err_out;   JDG
p = 0*(phi_cmd0 - phi) + 20*dpsidot + 0.0*psidot_err_out;

% limit max rollrate
if (p > phidotmax)
    p = phidotmax;
elseif (p < -phidotmax)
    p = -phidotmax;
end

% limit max bank angle
if (phi+p*0.1 > phimax)
    p = (phimax - phi)*10;
%elseif (phi-p*0.1 < -phimax)
    %p = (phimax - phi)*10;
elseif (phi+p*0.1 < -phimax)
    p = (-phimax - phi)*10;  %JDG - added negative on 9/17/07
end

== matlab function BasicAircraftDynamicsBlock/Basic Aircraft Dynamics/Pilot // Controller/compute q/Embedded MATLAB Function ==
  data: u input; phi_max output size=1; q_max input
function phi_max  = saturate_phi(u,q_max)
%#codegen

% This block supports the Embedded MATLAB subset.
% See the help menu for details. 
%
% This function keeps a running maximum bank angle.  The "pilot" controller
% in CASSATT will now sacrifice bank angle in order to maintain the correct
% vertical rate.
%
% Max bank angle is calculated using Equation 19 in "CASSATT v3.0 Dynamic
% Equations of Motion" (written 18 June 2007).  First, replace sin(phi)^2
% with (1-cos(phi)^2).  Second, solve the quadratic equation for cos(phi).
% Finally, calculate the maximum bank angle by taking arccos (and we also
% multiply by a small factor to create a "buffer" so the track doesn't
% jitter along the desired vertical rate).
%
% Creator: Dan Griffith
% Date: 6 October 2008


v = u(1);
theta = u(2);
phi = u(3);
a_cmd = u(4);
hdd_cmd = u(5);
g=32.2;

% Internally limit hdd so that when it is really big we don't force phi=0.
% This will create a nicer transient.  
hdd_cmd = min( hdd_cmd , v*q_max*cos(phi)*cos(theta) );

% calculate discriminant
sqrt_arg = v^2*q_max^2 - 4*g*a_cmd*sin(theta) + 4*g*hdd_cmd + ...
    4*g^2*cos(theta)^2;
if sqrt_arg<0
    phi_max = 10000;
    return
end

% calculate cos(phi)
cphi1 = ( -v*q_max + sqrt( sqrt_arg ) ) / (2*g*cos(theta));

% % JDG - I don't think I ever need this one.  It always results in an
% % imaginary angle
% cphi2 = ( -v*q_max - sqrt( sqrt_arg ) ) / (2*g*cos(theta))

if abs(cphi1) < 1
    phi_max  = acos( cphi1 )*.98; % add a small buffer to prevent jittering
else
    phi_max = 0; % well, we can't achieve rate, so set bank angle to zero and do our best
end

== matlab function BasicAircraftDynamicsBlock/Basic Aircraft Dynamics/Pilot // Controller/compute r1/Embedded MATLAB Function ==
  data: u input; y output
function y = fcn(u)
%#eml

if u==0
    y=1;
else
    y=2;
end
